simulink model "OpcConnectionTest"  (R2021a)
settings: Solver=VariableStepAuto  StartTime=0.0  StopTime=10.0  RelTol=1e-3
model workspace (MAT data in the model file):
  arraySize = 3
libraries: dspsrcs4 x2
settings Model: Creator=agustin  LastModifiedBy=agustin

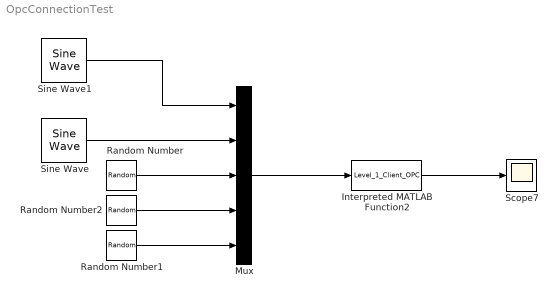
== system OpcConnectionTest ==
  Interpreted MATLAB Function2 : MATLABFcn  MATLABFcn=Level_1_Client_OPC  Output1D=off
  Mux : Mux  Inputs=5
  Random Number : RandomNumber  SampleTime=0.1
  Random Number1 : RandomNumber  SampleTime=0.1
  Random Number2 : RandomNumber  SampleTime=0.1
  Scope7 : Scope
  Sine Wave : dspsrcs4/Sine Wave  Amplitude=1  Frequency=100  Phase=0  SampleMode=Discrete  OutComplex=Real  CompMethod=Trigonometric fcn  TableSize=Speed  SampleTime=1/1000  SamplesPerFrame=1  ResetState=Restart at time zero  OutputFrames=off  dataType=double  wordLen=16  udDataType=sfix(16)  fracBitsMode=Best precision  numFracBits=15  OutDataTypeStr=double  LastOutDataTypeStr=double
  Sine Wave1 : dspsrcs4/Sine Wave  Amplitude=1  Frequency=100  Phase=0  SampleMode=Discrete  OutComplex=Real  CompMethod=Trigonometric fcn  TableSize=Speed  SampleTime=1/1000  SamplesPerFrame=1  ResetState=Restart at time zero  OutputFrames=off  dataType=double  wordLen=16  udDataType=sfix(16)  fracBitsMode=Best precision  numFracBits=15  OutDataTypeStr=double  LastOutDataTypeStr=double
  wires:
  Interpreted MATLAB Function2/1 -> Scope7/1
  Mux/1 -> Interpreted MATLAB Function2/1
  Sine Wave1/1 -> Mux/1
  Sine Wave/1 -> Mux/2
  Random Number1/1 -> Mux/5
  Random Number2/1 -> Mux/4
  Random Number/1 -> Mux/3
